simulink model "CSTRExampleControl"  (R2020a)
settings: Solver=FixedStepAuto  StartTime=0.0  StopTime=tfinal  FixedStep=step  MaxStep=10e-3  RelTol=1e-3
values from neighbouring files (symbols this model uses):
  Ca0 = 2.917496611031752    (= 2.91749661103)    [CSTRComputeOP.m]    (also in CSTRInit.m)
  Cb0 = 1.099991103606458    (= 1.09999110361)    [CSTRComputeOP.m]    (also in CSTRInit.m)
  k1 = 5/6    (= 0.833333333333)    [CSTRComputeOP.m]    (also in CSTRInit.m; CSTROP.m = param(1); sfun_CSTR.m = param(1))
  k2 = 5/3    (= 1.66666666667)    [CSTRComputeOP.m]    (also in CSTRInit.m; CSTROP.m = param(2); sfun_CSTR.m = param(2))
  k3 = 1/6    (= 0.166666666667)    [CSTRComputeOP.m]    (also in CSTRInit.m; CSTROP.m = param(3); sfun_CSTR.m = param(3))
  u0 = 60    [CSTRInit.m]
  V = 700    [CSTRComputeOP.m]    (also in CSTRInit.m; CSTROP.m = param(4); sfun_CSTR.m = param(4))
  y0 = 100/1.5714*Cb0    (= 70.000706606)    [CSTRInit.m]
undefined symbols (not defined in the file or in its folder): alpha, beta, gamma, Kp, Td, Ti
settings Model: Creator=david  LastModifiedBy=david

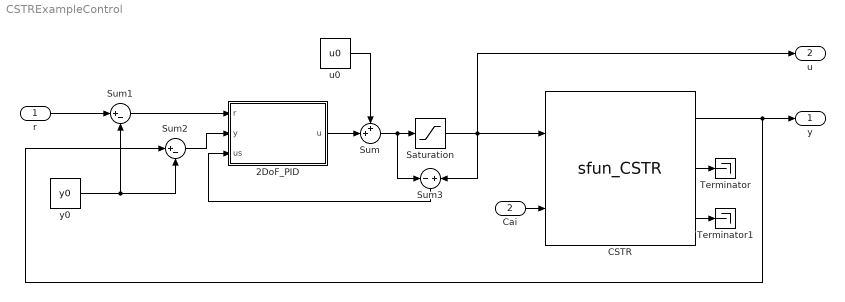
== system CSTRExampleControl ==
  r : Inport
  Cai : Inport  Port=2
  2DoF_PID : Subsystem  mask{Kp=Kp, Ti=Ti, Td=Td, alpha=alpha, beta=beta, gamma=gamma}
      mask DialogControl DescGroupVar Prompt: 2DoF PID controller
      mask DialogControl DescTextVar Prompt: Implementation of an industrial PID controller with two degrees of freedom
  CSTR : M-S-Function  FunctionName=sfun_CSTR  Parameters=|  mask{k1=k1, k2=k2, k3=k3, V=V, Ca0=Ca0, Cb0=Cb0}
      | [k1;
      | k2;
      | k3; V], [Ca0; Cb0]
      mask DialogControl DescGroupVar Prompt: Isothermal Van de Vusse reactor
      mask DialogControl DescTextVar Prompt: Model for the isothermal Van de Vusse reaction in a CSTR with constant volume
      mask Display:
      | port_label('output', 1, 'y')
      | port_label('output', 2, 'Ca')
      | port_label('output', 3, 'Cb')
      | port_label('input', 1, 'u')
      | port_label('input', 2, 'Cai')
      | image('VandeVusse.png')
  Saturation : Saturate  UpperLimit=100  LowerLimit=0
  Sum : Sum  Inputs=++|
  Sum1 : Sum  Inputs=|+-
  Sum2 : Sum  Inputs=|+-
  Sum3 : Sum  Inputs=-|+
  Terminator : Terminator
  Terminator1 : Terminator
  u0 : Constant  Value=u0
  y0 : Constant  Value=y0
  y : Outport
  u : Outport  Port=2
  wires:
  2DoF_PID/1(u) -> Sum/2
  Sum/1 -> Sum3/1, Saturation/1
  u0/1 -> Sum/1
  Sum1/1 -> 2DoF_PID/1(r)
  y0/1 -> Sum1/2, Sum2/2
  Sum2/1 -> 2DoF_PID/2(y)
  CSTR/1 -> y/1, Sum2/1
  CSTR/2 -> Terminator/1
  CSTR/3 -> Terminator1/1
  Saturation/1 -> u/1, Sum3/2, CSTR/1
  Sum3/1 -> 2DoF_PID/3(us)
  r/1 -> Sum1/1
  Cai/1 -> CSTR/2

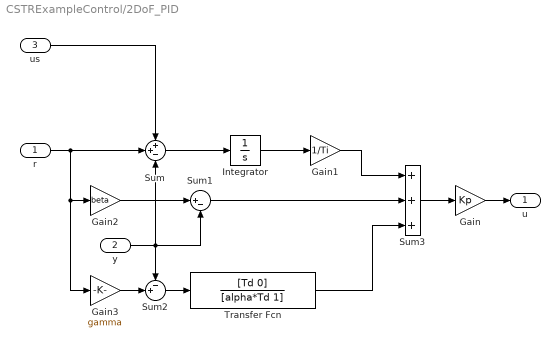
== system CSTRExampleControl/2DoF_PID ==
  r : Inport
  y : Inport  Port=2
  us : Inport  Port=3
  Gain : Gain  Gain=Kp
  Gain1 : Gain  Gain=1/Ti
  Gain2 : Gain  Gain=beta
  Gain3 : Gain  Gain=gamma
  Integrator : Integrator
  Sum : Sum  Inputs=++-
  Sum1 : Sum  Inputs=|+-
  Sum2 : Sum  Inputs=-+|
  Sum3 : Sum  Inputs=+++
  Transfer Fcn : TransferFcn  Numerator=[Td 0]  Denominator=[alpha*Td 1]
  u : Outport
  wires:
  y/1 -> Sum/3, Sum1/2, Sum2/1
  r/1 -> Sum/2, Gain3/1, Gain2/1
  Sum/1 -> Integrator/1
  Integrator/1 -> Gain1/1
  Gain2/1 -> Sum1/1
  Gain3/1 -> Sum2/2
  Sum2/1 -> Transfer Fcn/1
  Sum3/1 -> Gain/1
  Gain1/1 -> Sum3/1
  Sum1/1 -> Sum3/2
  Transfer Fcn/1 -> Sum3/3
  Gain/1 -> u/1
  us/1 -> Sum/1
